simulink model "rf"  (Simulink 7.1)
settings: Solver=ode45  StartTime=0.0  StopTime=tm  MaxStep=tr  RelTol=1e-3
values from neighbouring files (symbols this model uses):
  B = 52.2786    [mechanical_example.m]
  k = 113832    [mechanical_example.m]
  M = 12.5 * 0.45359237    (= 5.669904625)    [mechanical_example.m]
libraries: simulink x1
settings Model: Creator=christopher.rappa  LastModifiedBy=christopher.rappa
settings OptimizationCC: InlineInvariantSignals=on
settings DebuggingCC: SaveWithParameterizedLinksMsg=none  SignalResolutionControl=TryResolveAllWithWarning  MultiTaskDSMMsg=warning  MultiTaskCondExecSysMsg=none  StrictBusMsg=None
settings RTWCC: IncludeERTFirstTime=on
settings GRTTargetCC: TargetFcnLib=ansi_tfl_tmw.mat

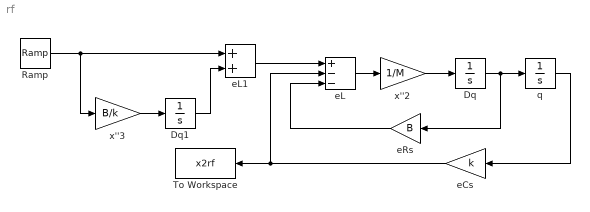
== system rf ==
  Dq : Integrator
  Dq1 : Integrator
  Ramp : simulink/Sources/Ramp  SystemSampleTime=-1  slope=1  start=0  X0=0
  To Workspace : ToWorkspace  VariableName=x2rf  SampleTime=-1  SaveFormat=Structure With Time
  eCs : Gain  Orientation=left  Gain=k  ParameterDataType=sfix(16)  ParameterScaling=2^0  OutDataType=sfix(16)  OutScaling=2^0
  eL : Sum  Inputs=+--  OutDataType=sfix(16)  OutScaling=2^-10
  eL1 : Sum  OutDataType=sfix(16)  OutScaling=2^-10
  eRs : Gain  Orientation=left  Gain=B  ParameterDataType=sfix(16)  ParameterScaling=2^0  OutDataType=sfix(16)  OutScaling=2^0
  q : Integrator
  x''2 : Gain  Gain=1/M  ParameterDataType=sfix(16)  ParameterScaling=2^0  OutDataType=sfix(16)  OutScaling=2^0
  x''3 : Gain  Gain=B/k  ParameterDataType=sfix(16)  ParameterScaling=2^0  OutDataType=sfix(16)  OutScaling=2^0
  wires:
  q/1 -> eCs/1
  eCs/1 -> eL/2, To Workspace/1
  Dq/1 -> q/1, eRs/1
  eRs/1 -> eL/3
  eL/1 -> x''2/1
  x''2/1 -> Dq/1
  Ramp/1 -> x''3/1, eL1/1
  eL1/1 -> eL/1
  x''3/1 -> Dq1/1
  Dq1/1 -> eL1/2
